simulink model "ss_plant_subj01"  (R2019a)
settings: Solver=ode14x  StartTime=0  StopTime=0.001  FixedStep=1e-5  RelTol=1e-3  EnableMultiTasking=on
model workspace (MAT data in the model file):
  Ankle_L_D = 1.86999822456
  Ankle_L_S = 0.0237763920936
  Ankle_R_D = 0.0588397140494
  Ankle_R_S = 0.739584271752
  BeginTimePlantModel = 0
  F_C = 0.0618
  F_H = 0.107
  F_I = 0.0129
  F_L = 0.2471
  F_M = 1.2499
  F_W = 0.11
  GRF_HD = 42097.5090581
  GRF_HS = 111995.804745
  GRF_VD = 23523.4518935
  GRF_VS = 88551.3661398
  HAT_I = 4.3688
  HAT_L = 0.549
  HAT_M = 58.9182
  HAT_a = 0.2
  HAT_b = 0.13
  Hip_L_D = 0.00120944164738
  Hip_L_S = 1.91959156409
  Hip_R_D = 0.00174333284727
  Hip_R_S = 0.483982271561
  Knee_L_D = 0.900041230997
  Knee_L_S = 0.0187606009115
  Knee_R_D = 0.0722123401531
  Knee_R_S = 0.0187606009115
  M : struct (value not decoded)
  S_I = 0.073
  S_L = 0.447
  S_M = 4.0083
  S_R1 = 0.06
  S_R2 = 0.08
  T_I = 0.2042
  T_L = 0.476
  T_M = 8.62
  T_R1 = 0.08
  T_R2 = 0.1
  bodymass = 86.2
  p_stance_ankle = 0.6904
  p_stance_hip = 14.7432
  p_stance_knee = -15.5578
  p_swing_ankle = -17.2995
  p_swing_hip = -9.1033
  p_swing_knee = -42.7648
  polyfit_stance_ankle = [23675.5212354 -31931.2429023 15252.5151968 -3621.5696911 268.973048302 -0.00762323811385]
  polyfit_swing_ankle = [-7183170.28304 10168157.4246 -5826762.40795 1748786.50975 -298844.069674 29567.8455925 -1567.7731554 24.418061318 1.56689555274]
  polyfit_swing_hip = [-184063768.654 261180473.575 -149801561.895 44513131.158 -7279965.6736 635960.536344 -25237.4588361 73.5247488612 22.0195049052]
  polyfit_swing_knee = [-121821446.299 173842986.405 -100273096.775 30000313.7158 -4970023.76394 451012.243214 -20836.4993451 353.694972881 6.37011560058]
  stance_hip_D = -0.2
  stance_hip_I = 0
  stance_hip_P = -2
  stance_knee_D = 0.1
  stance_knee_I = 0
  stance_knee_P = 1
  u_stance_ankle = [0 0 0 0 0 0]
  u_swing_ankle = [0 0 0 0 0 0]
  u_swing_hip = [0 0 0 0 0 0]
  u_swing_knee = [0 0 0 0 0 0]
  w_stance_ankle = 93.2507485327
  w_stance_hip = -74.2652398804
  w_stance_knee = -14.764511914
  w_swing_ankle = -75.522045152
  w_swing_hip = 188.938734782
  w_swing_knee = -287.34228095
values from neighbouring files (symbols this model uses):
  N = 3    [lagdmodel.m]
symbols that are objects in the model workspace (value not decoded): M
undefined symbols (not defined in the file or in its folder): X, Y, Z
libraries: nesl_utility x73, sm_lib x49, fl_lib x24, fl_ps_legacy_lib x16
(part 7 of 7)

== system ss_plant_subj01/Hip_R_Actuation/Hard_Stop_Hip_R/Rotational Simscape Intf (Library Block) ==
  Ideal Angular Velocity Source : fl_lib/Mechanical/Mechanical Sources/Ideal Angular Velocity Source
  Ideal Torque Sensor : fl_lib/Mechanical/Mechanical Sensors/Ideal Torque Sensor
  w : PMIOPort  Side=Left
  T : PMIOPort  Port=2  Side=Right
  R : PMIOPort  Port=3  Side=Left
  C : PMIOPort  Port=4  Side=Right
  connections:
  w/RConn1 -- Ideal Angular Velocity Source/RConn1
  T/RConn1 -- Ideal Torque Sensor/RConn2
  Ideal Torque Sensor/LConn1 -- Ideal Angular Velocity Source/RConn2
  R/RConn1 -- Ideal Angular Velocity Source/LConn1
  Ideal Torque Sensor/RConn1 -- C/RConn1

== system ss_plant_subj01/Knee_L_PID_control/Knee_L_Actuation1/Hard_Stop_Knee_L ==
  Mechanical Rotational Reference : fl_lib/Mechanical/Rotational Elements/Mechanical Rotational Reference
  Rotational Simscape Intf (Library Block) : Subsystem
  Rotational Hard Stop : fl_lib/Mechanical/Rotational Elements/Rotational Hard Stop  upper_bnd=upper_bound rad  lower_bnd=lower_bound rad  stiff_up=contact_stiffness N*m/rad  stiff_low=contact_stiffness N*m/rad  D_up=contact_damping N*m/(rad/s)  D_low=contact_damping N*m/(rad/s)  model=3  transition=0.001 rad  w_specify=off  w_priority=None  w=0 rad/s  w_nominal_specify=off  w_nominal_unit=rad/s  w_nominal_value=1  t_specify=off  t_priority=None  t=0 N*m  t_nominal_specify=off  t_nominal_unit=N*m  t_nominal_value=1  phi_specify=on  phi_priority=High  phi=initial_angular_position rad  phi_nominal_specify=off  phi_nominal_unit=rad  phi_nominal_value=1
      settings: SourceProductName=Simscape  SourceProductBaseCode=SS
  T : PMIOPort  Side=Right
  w : PMIOPort  Port=2  Side=Left
  connections:
  Rotational Simscape Intf (Library Block)/RConn1 -- T/RConn1
  w/RConn1 -- Rotational Simscape Intf (Library Block)/LConn1
  Rotational Hard Stop/RConn1 -- Rotational Simscape Intf (Library Block)/RConn2
  Mechanical Rotational Reference/LConn1 -- Rotational Hard Stop/LConn1 -- Rotational Simscape Intf (Library Block)/LConn2

== system ss_plant_subj01/Knee_R_Actuation/Hard_Stop_Knee_L1/Rotational Simscape Intf (Library Block) ==
  Ideal Angular Velocity Source : fl_lib/Mechanical/Mechanical Sources/Ideal Angular Velocity Source
  Ideal Torque Sensor : fl_lib/Mechanical/Mechanical Sensors/Ideal Torque Sensor
  w : PMIOPort  Side=Left
  T : PMIOPort  Port=2  Side=Right
  R : PMIOPort  Port=3  Side=Left
  C : PMIOPort  Port=4  Side=Right
  connections:
  Ideal Torque Sensor/RConn1 -- C/RConn1
  R/RConn1 -- Ideal Angular Velocity Source/LConn1
  Ideal Torque Sensor/LConn1 -- Ideal Angular Velocity Source/RConn2
  T/RConn1 -- Ideal Torque Sensor/RConn2
  w/RConn1 -- Ideal Angular Velocity Source/RConn1

== system ss_plant_subj01/Hip_L_PID_Control/Hip_L_Actuation1/Hard_Stop_Hip_L/Rotational Simscape Intf (Library Block) ==
  Ideal Angular Velocity Source : fl_lib/Mechanical/Mechanical Sources/Ideal Angular Velocity Source
  Ideal Torque Sensor : fl_lib/Mechanical/Mechanical Sensors/Ideal Torque Sensor
  w : PMIOPort  Side=Left
  T : PMIOPort  Port=2  Side=Right
  R : PMIOPort  Port=3  Side=Left
  C : PMIOPort  Port=4  Side=Right
  connections:
  w/RConn1 -- Ideal Angular Velocity Source/RConn1
  T/RConn1 -- Ideal Torque Sensor/RConn2
  Ideal Torque Sensor/LConn1 -- Ideal Angular Velocity Source/RConn2
  R/RConn1 -- Ideal Angular Velocity Source/LConn1
  Ideal Torque Sensor/RConn1 -- C/RConn1

== system ss_plant_subj01/Knee_L_PID_control/Knee_L_Actuation1/Hard_Stop_Knee_L/Rotational Simscape Intf (Library Block) ==
  Ideal Angular Velocity Source : fl_lib/Mechanical/Mechanical Sources/Ideal Angular Velocity Source
  Ideal Torque Sensor : fl_lib/Mechanical/Mechanical Sensors/Ideal Torque Sensor
  w : PMIOPort  Side=Left
  T : PMIOPort  Port=2  Side=Right
  R : PMIOPort  Port=3  Side=Left
  C : PMIOPort  Port=4  Side=Right
  connections:
  Ideal Torque Sensor/RConn1 -- C/RConn1
  R/RConn1 -- Ideal Angular Velocity Source/LConn1
  Ideal Torque Sensor/LConn1 -- Ideal Angular Velocity Source/RConn2
  T/RConn1 -- Ideal Torque Sensor/RConn2
  w/RConn1 -- Ideal Angular Velocity Source/RConn1
